simulink model "P_2_1_d_Predacio_modell"  (R2021b)
settings: Solver=VariableStepAuto  StartTime=0.0  StopTime=10.0  MaxStep=0.01  RelTol=1e-3
settings Model: Creator=davidpaksi  LastModifiedBy=davidpaksi

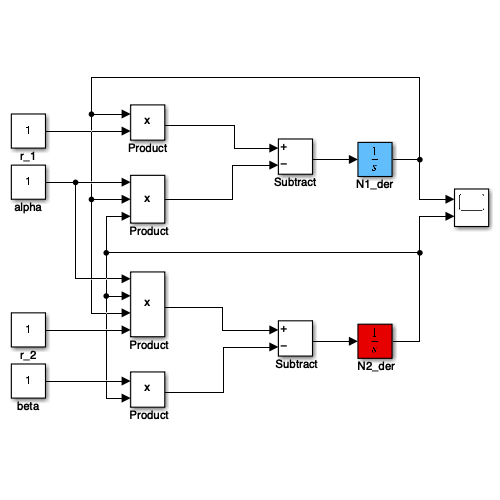
[thumbnail: Simulink's stored preview of the top-level diagram]
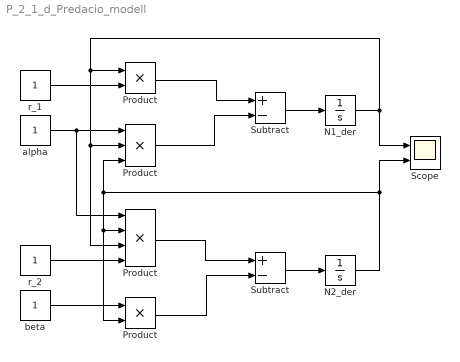
== system P_2_1_d_Predacio_modell ==
  "   Product  " : Product
  "  Product " : Product  Inputs=4
  " N1_der " : Integrator  InitialCondition=2
  " N2_der" : Integrator  InitialCondition=1
  " Product" : Product  Inputs=3
  " Product " : Product
  " Subtract" : Sum  Inputs=+-
  " Subtract " : Sum  Inputs=+-
  Scope : Scope  NumInputPorts=2
  alpha : Constant
  beta : Constant
  r_1 : Constant
  r_2 : Constant
  wires:
  " Subtract "/1 -> " N1_der "/1
  " Product "/1 -> " Subtract "/1
  " Product"/1 -> " Subtract "/2
  r_1/1 -> " Product "/2
  " N1_der "/1 -> " Product "/1, " Product"/2, "  Product "/3, Scope/1
  alpha/1 -> " Product"/1, "  Product "/1
  " N2_der"/1 -> Scope/2, "   Product  "/2, "  Product "/2, " Product"/3
  " Subtract"/1 -> " N2_der"/1
  "  Product "/1 -> " Subtract"/1
  "   Product  "/1 -> " Subtract"/2
  r_2/1 -> "  Product "/4
  beta/1 -> "   Product  "/1
